simulink model "zuoye4"  (R2018b)
settings: Solver=ode45  StartTime=0.0  StopTime=8  RelTol=1e-3
settings Model: Creator=12732  LastModifiedBy=12732
settings DataIOCC: SaveFormat=Array
settings DebuggingCC: LibraryContextMissingDiagnostic=none
settings SFSimCC: SimUseLocalCustomCode=off
settings RTWCC: RTWUseLocalCustomCode=off

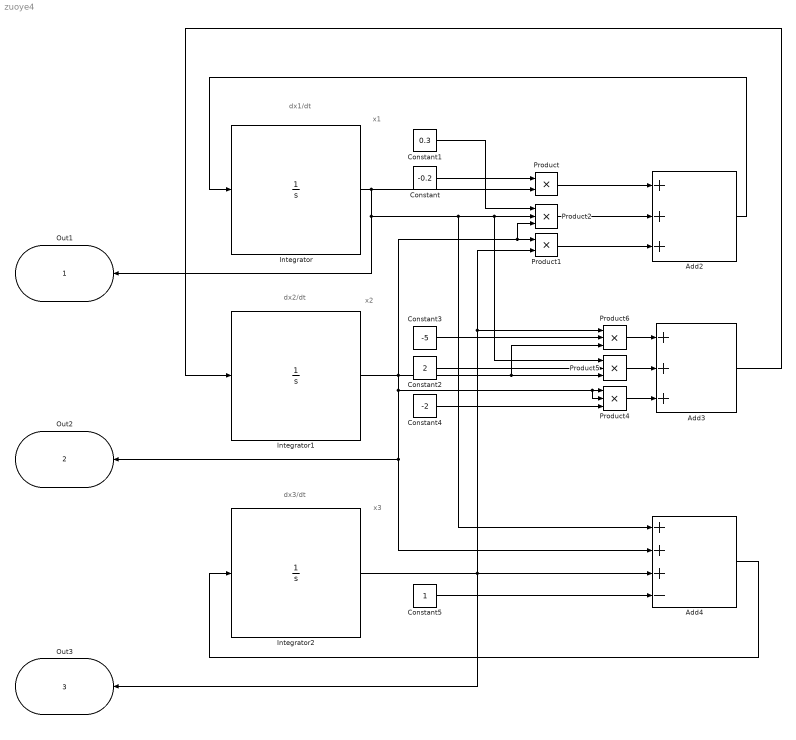
== system zuoye4 ==
  note: dx3/dt
  note: dx2/dt
  note: x3
  note: x2
  note: x1
  note: dx1/dt
  Add2 : Sum  Inputs=+++
  Add3 : Sum  Inputs=+++
  Add4 : Sum  Inputs=+++-
  Constant : Constant  Value=-0.2
  Constant1 : Constant  Value=0.3
  Constant2 : Constant  Value=2
  Constant3 : Constant  Value=-5
  Constant4 : Constant  Value=-2
  Constant5 : Constant
  Integrator : Integrator  InitialCondition=0.8
  Integrator1 : Integrator  InitialCondition=0.1
  Integrator2 : Integrator  InitialCondition=0.1
  Product : Product
  Product1 : Product
  Product{2,4..6} (4 alike) : Product  Inputs=3
  Out1 : Outport
  Out2 : Outport  Port=2
  Out3 : Outport  Port=3
  wires:
  Constant3/1 -> Product6/2
  Add2/1 -> Integrator/1
  Add3/1 -> Integrator1/1
  Constant4/1 -> Product4/3
  Constant5/1 -> Add4/4
  Product2/1 -> Add2/2
  Constant2/1 -> Product5/2
  Product5/1 -> Add3/2
  Product/1 -> Add2/1
  Integrator2/1 -> Out3/1, Product1/2, Product6/1, Add4/3
  Product1/1 -> Add2/3
  Integrator1/1 -> Product1/1, Product2/3, Out2/1, Add4/2, Product4/2, Product4/1, Product6/3, Product5/3
  Constant1/1 -> Product2/1
  Constant/1 -> Product/1
  Add4/1 -> Integrator2/1
  Product6/1 -> Add3/1
  Integrator/1 -> Out1/1, Product2/2, Product5/1, Add4/1, Product/2
  Product4/1 -> Add3/3
